simulink model "open_loop_dyn"  (R2022a)
settings: Solver=ode45  StartTime=0.0  StopTime=10.0  FixedStep=0.01  RelTol=1e-3
undefined symbols (not defined in the file): dt, f, fx, fy, fz, nx, ny, nz, tau, xee0, xee_dot_0
settings Model: Creator=charl  LastModifiedBy=charl

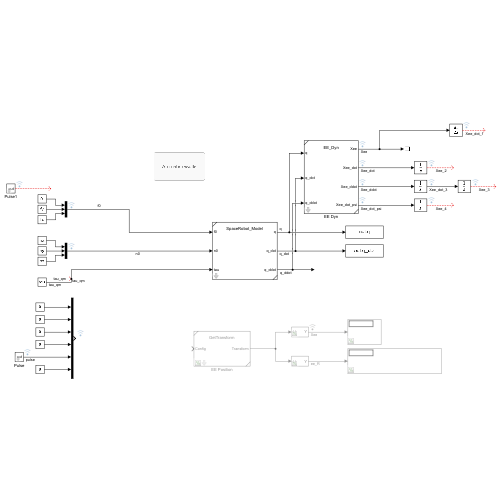
[thumbnail: Simulink's stored preview of the top-level diagram]
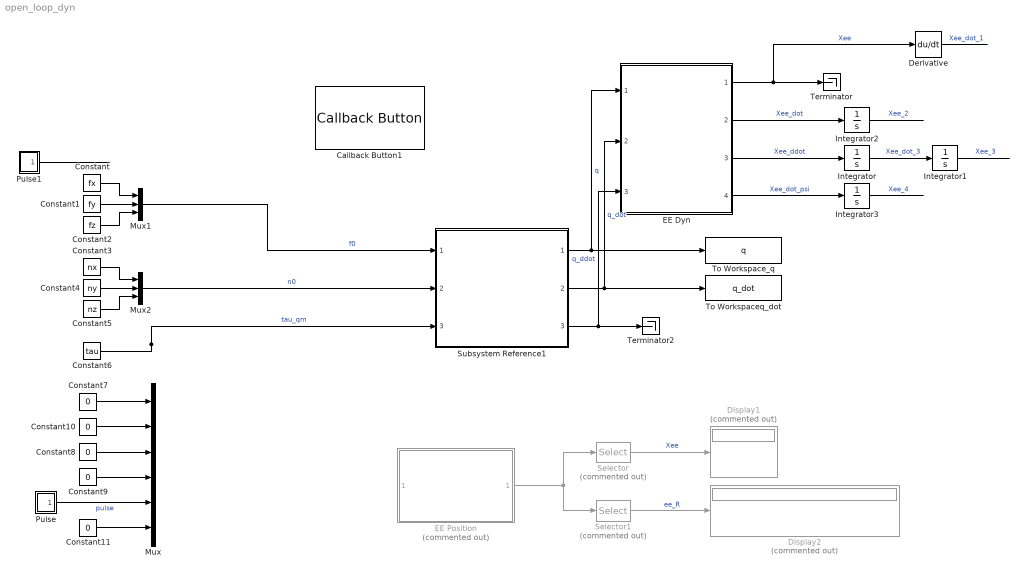
== system open_loop_dyn ==
  Callback Button1 : CallbackButton  ButtonText=Animate results
      settings: ClickFcn=|
      | close all
      | sr.animate(out.q, 'fps', 17, 'rate', 1);
  Constant : Constant  Value=fx
  Constant1 : Constant  Value=fy
  Constant{7..11} (5 alike) : Constant  Value=0
  Constant2 : Constant  Value=fz
  Constant3 : Constant  Value=nx
  Constant4 : Constant  Value=ny
  Constant5 : Constant  Value=nz
  Constant6 : Constant  Value=tau
  Derivative : Derivative
  Display1 : Display  Commented=on
  Display2 : Display  Commented=on
  EE Dyn : Subsystem  ReferencedSubsystem=EE_Dyn  spaceRobot=sr  Xee0=0
  EE Position : Subsystem  Commented=on  ReferencedSubsystem=GetTransform  spaceRobot=sr  sourceBody=endeffector  targetBody=inertial  SimulateUsing=Interpreted execution
  Integrator : Integrator  InitialCondition=xee_dot_0
  Integrator1 : Integrator  InitialCondition=xee0
  Integrator2 : Integrator  InitialCondition=xee0
  Integrator3 : Integrator  InitialCondition=xee0
  Mux : Mux  Inputs=6
  Mux1 : Mux  Inputs=3
  Mux2 : Mux  Inputs=3
  Pulse : Subsystem  mask{t_start=1, f=f, dt=dt}
      mask prompts: t_start "Start Time"; f "Amplitude"; dt "Width"
  Pulse1 : Subsystem  mask{t_start=1, f=f, dt=dt}
      mask prompts: t_start "Start Time"; f "Amplitude"; dt "Width"
  Selector : Selector  Commented=on  NumberOfDimensions=2  InputPortWidth=[4 4]  IndexOptions=Index vector (dialog),Index vector (dialog)  Indices=[1:3],4  OutputSizes=1,1
  Selector1 : Selector  Commented=on  NumberOfDimensions=2  InputPortWidth=[4 4]  IndexOptions=Index vector (dialog),Index vector (dialog)  Indices=[1:3],[1:3]  OutputSizes=1,1
  Subsystem Reference1 : Subsystem  ReferencedSubsystem=SpaceRobot_Model  spaceRobot=sr  jointCstr=off  q_0=q_0  q_dot_0=q_dot_0
  Terminator : Terminator
  Terminator2 : Terminator
  To Workspace_q : ToWorkspace  VariableName=q  SaveFormat=Timeseries  SampleTime=-1
  To Workspaceq_dot : ToWorkspace  VariableName=q_dot  SaveFormat=Timeseries  SampleTime=-1
  wires:
  Mux2/1 -> Subsystem Reference1/2  "n0"
  Subsystem Reference1/1 -> EE Dyn/1, To Workspace_q/1  "q"
  Subsystem Reference1/2 -> EE Dyn/2, To Workspaceq_dot/1  "q_dot"
  Mux1/1 -> Subsystem Reference1/1  "f0"
  Constant1/1 -> Mux1/2
  Constant2/1 -> Mux1/3
  Constant4/1 -> Mux2/2
  Pulse1/1(out) -> ?
  Constant5/1 -> Mux2/3
  Constant7/1 -> Mux/1
  Constant/1 -> Mux1/1
  Constant3/1 -> Mux2/1
  Selector1/1 -> Display2/1  "ee_R"
  Selector/1 -> Display1/1  "Xee"
  EE Position/1 -> Selector1/1, Selector/1
  EE Dyn/1 -> Derivative/1, Terminator/1  "Xee"
  EE Dyn/2 -> Integrator2/1  "Xee_dot"
  Subsystem Reference1/3 -> Terminator2/1, EE Dyn/3  "q_ddot"
  EE Dyn/3 -> Integrator/1  "Xee_ddot"
  Constant8/1 -> Mux/3
  Constant9/1 -> Mux/4
  Constant11/1 -> Mux/6
  Pulse/1(out) -> Mux/5  "pulse"
  Constant10/1 -> Mux/2
  Constant6/1 -> Subsystem Reference1/3  "tau_qm"
  Integrator/1 -> Integrator1/1  "Xee_dot_3"
  Integrator1/1 -> ?  "Xee_3"
  Integrator2/1 -> ?  "Xee_2"
  Integrator3/1 -> ?  "Xee_4"
  EE Dyn/4 -> Integrator3/1  "Xee_dot_psi"
  Derivative/1 -> ?  "Xee_dot_1"

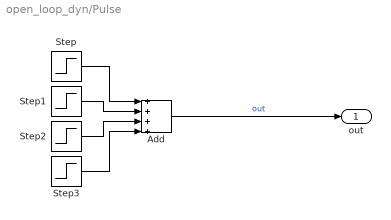
== system open_loop_dyn/Pulse ==
  Add : Sum  Inputs=++++
  Step : Step  Time=t_start  After=f  SampleTime=0
  Step1 : Step  Time=t_start+dt  After=-f  SampleTime=0
  Step2 : Step  Time=t_start+2*dt  After=-f  SampleTime=0
  Step3 : Step  Time=t_start+3*dt  After=f  SampleTime=0
  out : Outport
  wires:
  Step3/1 -> Add/4
  Add/1 -> out/1  "out"
  Step2/1 -> Add/3
  Step1/1 -> Add/2
  Step/1 -> Add/1

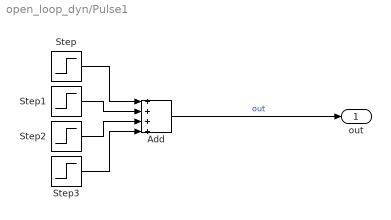
== system open_loop_dyn/Pulse1 ==
  Add : Sum  Inputs=++++
  Step : Step  Time=t_start  After=f  SampleTime=0
  Step1 : Step  Time=t_start+dt  After=-f  SampleTime=0
  Step2 : Step  Time=t_start+2*dt  After=-f  SampleTime=0
  Step3 : Step  Time=t_start+3*dt  After=f  SampleTime=0
  out : Outport
  wires:
  Step3/1 -> Add/4
  Add/1 -> out/1  "out"
  Step2/1 -> Add/3
  Step1/1 -> Add/2
  Step/1 -> Add/1
